simulink model "main_sim"  (R2024b)
settings: Solver=ode15s  StartTime=0.0  StopTime=t_sim  RelTol=1e-3
InitFcn:
  | rng('shuffle');
values from neighbouring files (symbols this model uses):
  accel_bias_instability = 9.8*40e-6    (= 0.000392)    [main.m]
  accel_PSD = accel_noise_power^2    (= 4.70596e-07)    [main.m]
  EA_0 = deg2rad([-2.83 -9.89 149]')    [Choi_SimulinkScript.m]    (also in SADS_UKF_Script.m = deg2rad([10 3 6]'); main.m = deg2rad([-8, 15, 0]'))
  g_N = [0 0 -9.81]    [Choi_SimulinkScript.m]    (also in SADS_UKF_Script.m; main.m)
  gyro_bias_instability = (pi/180)*(6/3600)    (= 2.90888208666e-05)    [main.m]
  gyro_PSD = gyro_noise_power^2    (= 2.74155703361e-09)    [main.m]
  J_0 = [1.815  -0.014 0.004 ... (first row only)    [Choi_SimulinkScript.m]    (also in LSR_sim.m = S.J_0; main.m)
  K_I = gainScale*5    (= 2.5)    [Choi_SimulinkScript.m]    (also in main.m)
  K_omega = gainScale*1    (= 0.5)    [Choi_SimulinkScript.m]    (also in main.m)
  k_p = 0.001    [Choi_SimulinkScript.m]
  K_q = gainScale*1    (= 0.5)    [Choi_SimulinkScript.m]    (also in main.m)
  L = [sample_time*(J_0\eye(3)), zeros(3,4) ... (first row only)    [main.m]
  m_s = 29    [Choi_SimulinkScript.m]    (also in LSR_sim.m = S.m_s; SADS_UKF_Script.m; main.m)
  omega_0 = [0 0.00 0.06]'    [Choi_SimulinkScript.m]    (also in SADS_UKF_Script.m = [0 0.00 0.05]'; main.m)
  P_0 = diag([1e-6 1e-6 1e-6 1e-6 1e-6 1e-6 1e-6 1e-6])    [SADS_UKF_Script.m]    (also in main.m = diag([1e-6 1e-6 1e-6 1e-6 1e-6 1e-6 1e-6]))
  Q = diag([5e-5 5e-5 5e-5 4e-12 4e-12 4e-12 4e-12 5e-6])    [SADS_UKF_Script.m]    (also in main.m = diag([5e-5 5e-5 5e-5 4e-11 4e-11 4e-11 4e-11]))
  q_0 = eul2quat(EA_0',"XYZ")'    [Choi_SimulinkScript.m]    (also in SADS_UKF_Script.m; main.m)
  q_d = [1 0 0 0]'    [Choi_SimulinkScript.m]    (also in main.m)
  R = diag([0.005 0.005 0.005].^2)    [SADS_UKF_Script.m]    (also in main.m)
  r_0 = [4*10^-3, 2*10^-3 ,-2*10^-2]'    [Choi_SimulinkScript.m]    (also in SADS_UKF_Script.m = [-0.003 0.006 -0.010]'; main.m = [0 0 0]')
  r_hat_0 = [0 0 -0.1]'    [Choi_SimulinkScript.m]
  r_imu_b = [0.1524, 0, 0.1524]    [main.m]
  sample_time = 1/sample_rate    (= 0.04)    [SADS_UKF_Script.m]    (also in main.m = 0.1)
  x_0 = [omega_0; q_0; 0]    [SADS_UKF_Script.m]
undefined symbols (not defined in the file or in its folder): A_pinv, A_truth, DiscIntNeverNeededParam, Gamma, gamma, h_d_amp, h_d_amp_LSR, h_d_period, h_d_period_LSR, h_d_phase, h_d_phase_LSR, H_ukf, I_wheel, Kappa, Kd_FSFB, Kp_FSFB, P_0_ukf, Q_ukf, R_ukf, tau_delay, x_0_ukf
libraries: simulink x6, matrix_library x4, sharedtransform x2, simulink_extras x1
settings Model: Creator=camer  LastModifiedBy=camer

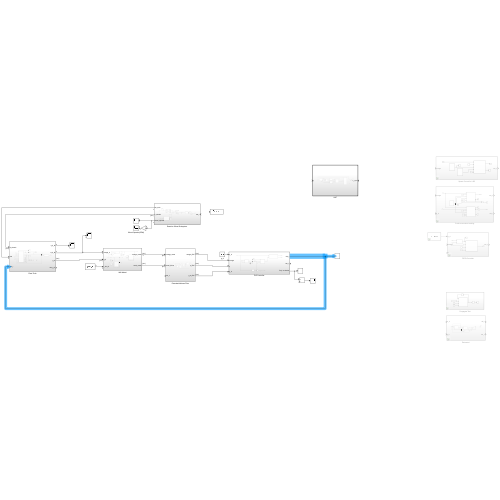
[thumbnail: Simulink's stored preview of the top-level diagram]
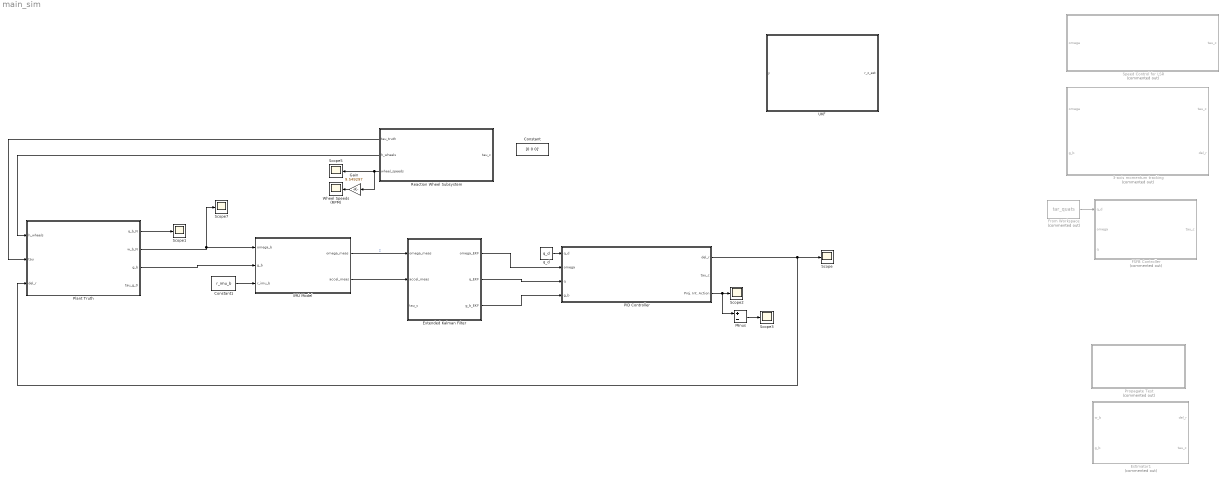
== system main_sim ==
  3-axis momentum tracking : Subsystem  Commented=on
  Constant : Constant  Value=[0 0 0]'
  Constant1 : Constant  Value=r_imu_b
  Estimator1 : Subsystem  Commented=on
  Extended Kalman Filter : Subsystem
  FSFB Controller : Subsystem  Commented=on
  From Workspace : FromWorkspace  Commented=on  VariableName=tar_quats
  Gain : Gain  Gain=9.549297
  IMU Model : Subsystem
  Minus : Sum  Inputs=+-
  PID Controller : Subsystem
  Plant Truth : Subsystem
  Propagate Test : Subsystem  Commented=on
  Reaction Wheel Subsystem : Subsystem
  Scope{,1..3,5,7} (6 alike) : Scope
  Speed Control for LSR : Subsystem  Commented=on
  UKF : Subsystem  TreatAsAtomicUnit=on
  Wheel Speeds (RPM) : Scope
  q_d : Constant  Value=q_d
  wires:
  IMU Model/1(omega_meas) -> Extended Kalman Filter/1(omega_meas)  "z"
  Constant1/1 -> IMU Model/3(r_imu_b)
  IMU Model/2(accel_meas) -> Extended Kalman Filter/2(accel_meas)
  From Workspace/1 -> FSFB Controller/1(q_d)
  Plant Truth/1(q_b_N) -> Scope1/1
  Reaction Wheel Subsystem/3(wheel_speeds) -> Scope5/1, Gain/1
  Reaction Wheel Subsystem/1(tau_truth) -> Plant Truth/2(tau)
  Plant Truth/2(w_b_N) -> Scope7/1, IMU Model/1(omega_b)
  Plant Truth/3(g_b) -> IMU Model/2(g_b)
  Reaction Wheel Subsystem/2(h_wheels) -> Plant Truth/1(h_wheels)
  Gain/1 -> Wheel Speeds (RPM)/1
  PID Controller/1(del_r) -> Plant Truth/3(del_r), Scope/1
  PID Controller/3(Proj. Int. Action) -> Minus/1, Scope2/1
  Minus/1 -> Scope3/1
  q_d/1 -> PID Controller/1(q_d)
  Extended Kalman Filter/1(omega_EKF) -> PID Controller/2(omega)
  Extended Kalman Filter/2(q_EKF) -> PID Controller/3(q)
  Extended Kalman Filter/3(g_b_EKF) -> PID Controller/4(g_b)

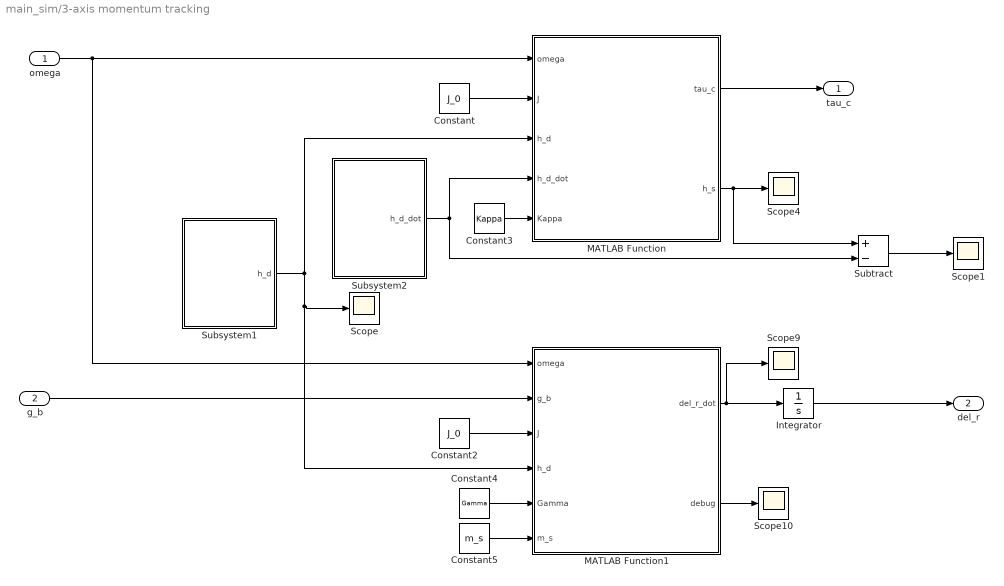
== system main_sim/3-axis momentum tracking ==
  omega : Inport
  g_b : Inport  Port=2
  Constant : Constant  Value=J_0
  Constant2 : Constant  Value=J_0
  Constant3 : Constant  Value=Kappa
  Constant4 : Constant  Value=Gamma
  Constant5 : Constant  Value=m_s
  Integrator : Integrator  InitialCondition=[0 0 0]'
  MATLAB Function : MATLAB Function  TreatAsAtomicUnit=on
  MATLAB Function1 : MATLAB Function  TreatAsAtomicUnit=on
  Scope{,1,4,9..10} (5 alike) : Scope
  Subsystem1 : Subsystem
  Subsystem2 : Subsystem
  Subtract : Sum  Inputs=+-
  tau_c : Outport
  del_r : Outport  Port=2
  wires:
  g_b/1 -> MATLAB Function1/2(g_b)
  Constant/1 -> MATLAB Function/2(J)
  MATLAB Function1/2(debug) -> Scope10/1
  MATLAB Function1/1(del_r_dot) -> Integrator/1, Scope9/1
  Constant2/1 -> MATLAB Function1/3(J)
  MATLAB Function/1(tau_c) -> tau_c/1
  MATLAB Function/2(h_s) -> Subtract/1, Scope4/1
  Constant4/1 -> MATLAB Function1/5(Gamma)
  Constant5/1 -> MATLAB Function1/6(m_s)
  omega/1 -> MATLAB Function1/1(omega), MATLAB Function/1(omega)
  Constant3/1 -> MATLAB Function/5(Kappa)
  Integrator/1 -> del_r/1
  Subsystem2/1(h_d_dot) -> Subtract/2, MATLAB Function/4(h_d_dot)
  Subsystem1/1(h_d) -> Scope/1, MATLAB Function1/4(h_d), MATLAB Function/3(h_d)
  Subtract/1 -> Scope1/1

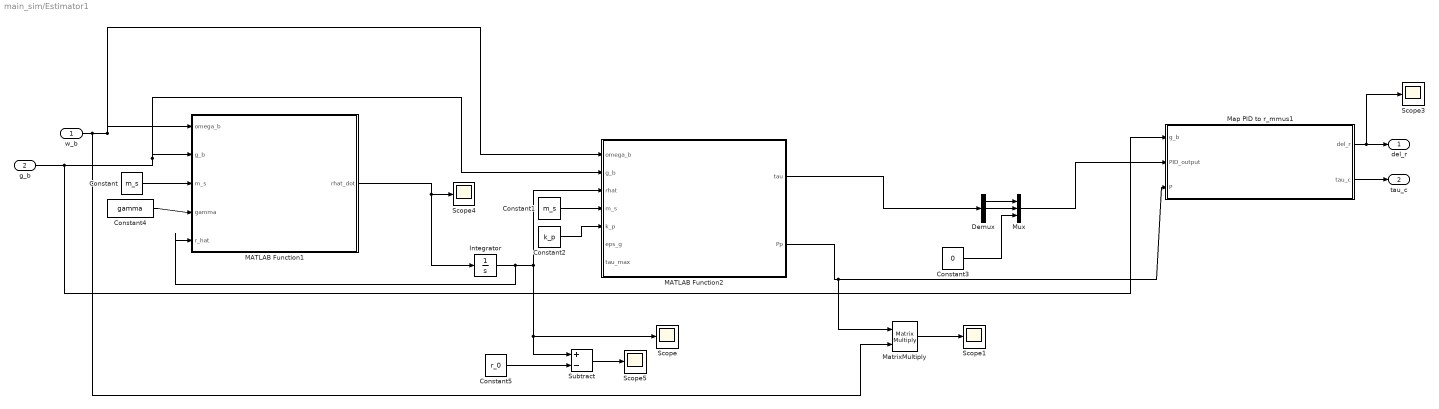
== system main_sim/Estimator1 ==
  w_b : Inport
  g_b : Inport  Port=2
  Constant : Constant  Value=m_s
  Constant1 : Constant  Value=m_s
  Constant2 : Constant  Value=k_p
  Constant3 : Constant  Value=0
  Constant4 : Constant  Value=gamma
  Constant5 : Constant  Value=r_0
  Demux : Demux  Outputs=3
  Integrator : Integrator  InitialCondition=r_hat_0
  MATLAB Function1 : MATLAB Function  TreatAsAtomicUnit=on
  MATLAB Function2 : MATLAB Function  TreatAsAtomicUnit=on
  Map PID to r_mmus1 : Subsystem
  MatrixMultiply : Product  Multiplication=Matrix(*)
  Mux : Mux  Inputs=3
  Scope{,1,3..5} (5 alike) : Scope
  Subtract : Sum  Inputs=+-
  del_r : Outport
  tau_c : Outport  Port=2
  wires:
  g_b/1 -> Map PID to r_mmus1/1(g_b), MATLAB Function2/2(g_b), MATLAB Function1/2(g_b)
  Constant/1 -> MATLAB Function1/3(m_s)
  MATLAB Function1/1(rhat_dot) -> Scope4/1, Integrator/1
  Integrator/1 -> MATLAB Function1/5(r_hat), Subtract/1, Scope/1, MATLAB Function2/3(rhat)
  Constant1/1 -> MATLAB Function2/4(m_s)
  Constant2/1 -> MATLAB Function2/5(k_p)
  MATLAB Function2/1(tau) -> Demux/1
  Demux/1 -> Mux/1
  Constant3/1 -> Mux/3
  Demux/2 -> Mux/2
  Map PID to r_mmus1/1(del_r) -> Scope3/1, del_r/1
  w_b/1 -> MatrixMultiply/2, MATLAB Function1/1(omega_b), MATLAB Function2/1(omega_b)
  Constant4/1 -> MATLAB Function1/4(gamma)
  Map PID to r_mmus1/2(tau_c) -> tau_c/1
  MATLAB Function2/2(Pp) -> MatrixMultiply/1, Map PID to r_mmus1/3(P)
  MatrixMultiply/1 -> Scope1/1
  Constant5/1 -> Subtract/2
  Subtract/1 -> Scope5/1
  Mux/1 -> Map PID to r_mmus1/2(PID_output)

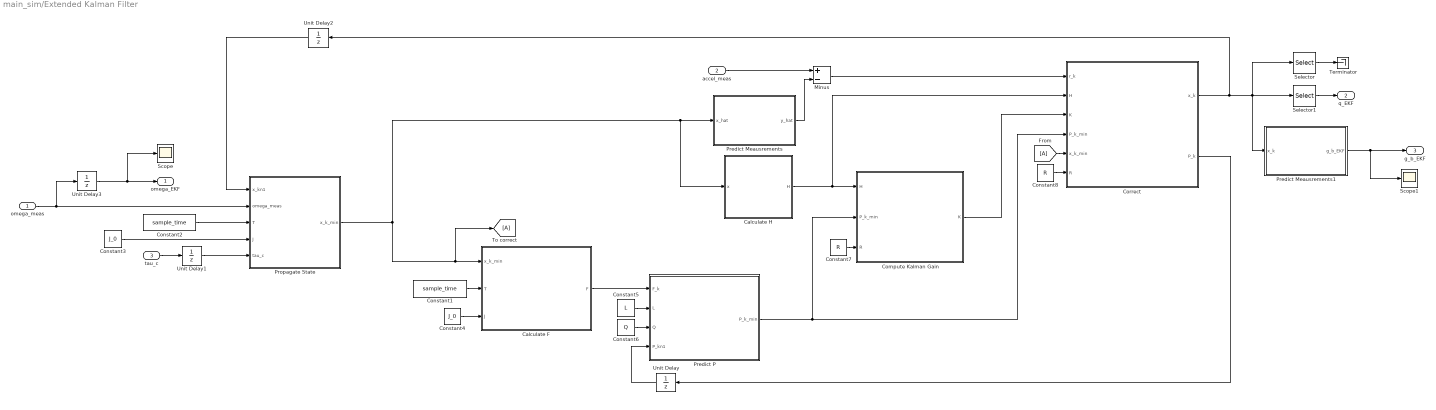
== system main_sim/Extended Kalman Filter ==
  omega_meas : Inport
  accel_meas : Inport  Port=2
  tau_c : Inport  Port=3
  Calculate F : MATLAB Function  TreatAsAtomicUnit=on
  Calculate H : MATLAB Function  TreatAsAtomicUnit=on
  Compute Kalman Gain : MATLAB Function  TreatAsAtomicUnit=on
  Constant1 : Constant  Value=sample_time
  Constant2 : Constant  Value=sample_time
  Constant3 : Constant  Value=J_0
  Constant4 : Constant  Value=J_0
  Constant5 : Constant  Value=L
  Constant6 : Constant  Value=Q
  Constant7 : Constant  Value=R
  Constant8 : Constant  Value=R
  Correct : MATLAB Function  TreatAsAtomicUnit=on
  From : From
  Minus : Sum  Inputs=+-
  Predict Meausrements : MATLAB Function  TreatAsAtomicUnit=on
  Predict Meausrements1 : MATLAB Function  TreatAsAtomicUnit=on
  Predict P : MATLAB Function  TreatAsAtomicUnit=on
  Propagate State : MATLAB Function  TreatAsAtomicUnit=on
  Scope : Scope
  Scope1 : Scope
  Selector : Selector  InputPortWidth=7  IndexOptions=Index vector (dialog)  Indices=[1 2 3]  OutputSizes=1
  Selector1 : Selector  InputPortWidth=7  IndexOptions=Index vector (dialog)  Indices=[4 5 6 7]  OutputSizes=1
  Terminator : Terminator
  To correct : Goto
  Unit Delay : UnitDelay  InitialCondition=P_0  SampleTime=sample_time  HasFrameUpgradeWarning=on
  Unit Delay1 : UnitDelay  InitialCondition=[0 0 0]'  SampleTime=-1  HasFrameUpgradeWarning=on
  Unit Delay2 : UnitDelay  InitialCondition=x_0  SampleTime=sample_time  HasFrameUpgradeWarning=on
  Unit Delay3 : UnitDelay  InitialCondition=[0 0 0]'  SampleTime=-1  HasFrameUpgradeWarning=on
  omega_EKF : Outport
  q_EKF : Outport  Port=2
  g_b_EKF : Outport  Port=3
  wires:
  Constant3/1 -> Propagate State/4(J)
  Propagate State/1(x_k_min) -> Calculate H/1(x), Predict Meausrements/1(x_hat), To correct/1, Calculate F/1(x_k_min)
  Unit Delay2/1 -> Propagate State/1(x_kn1)
  Constant2/1 -> Propagate State/3(T)
  Constant1/1 -> Calculate F/2(T)
  Constant4/1 -> Calculate F/3(J)
  Calculate F/1(F) -> Predict P/1(F_k)
  Unit Delay/1 -> Predict P/4(P_kn1)
  Constant5/1 -> Predict P/2(L)
  Constant6/1 -> Predict P/3(Q)
  accel_meas/1 -> Minus/1
  Predict Meausrements/1(y_hat) -> Minus/2
  Minus/1 -> Correct/1(r_k)
  Calculate H/1(H) -> Correct/2(H), Compute Kalman Gain/1(H)
  Predict P/1(P_k_min) -> Compute Kalman Gain/2(P_k_min), Correct/4(P_k_min)
  Constant7/1 -> Compute Kalman Gain/3(R)
  Compute Kalman Gain/1(K) -> Correct/3(K)
  Constant8/1 -> Correct/6(R)
  Correct/2(P_k) -> Unit Delay/1
  From/1 -> Correct/5(x_k_min)
  omega_meas/1 -> Propagate State/2(omega_meas), Unit Delay3/1
  Correct/1(x_k) -> Selector/1, Selector1/1, Predict Meausrements1/1(x_k), Unit Delay2/1
  Predict Meausrements1/1(g_b_EKF) -> Scope1/1, g_b_EKF/1
  Selector/1 -> Terminator/1
  Selector1/1 -> q_EKF/1
  tau_c/1 -> Unit Delay1/1
  Unit Delay1/1 -> Propagate State/5(tau_c)
  Unit Delay3/1 -> Scope/1, omega_EKF/1

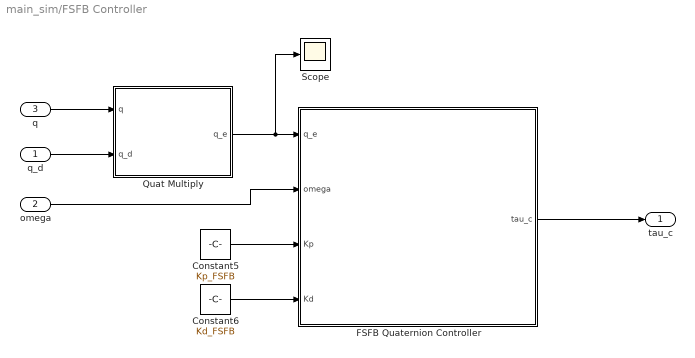
== system main_sim/FSFB Controller ==
  q_d : Inport
  omega : Inport  Port=2
  q : Inport  Port=3
  Constant5 : Constant  Value=Kp_FSFB
  Constant6 : Constant  Value=Kd_FSFB
  FSFB Quaternion Controller : MATLAB Function  TreatAsAtomicUnit=on
  Quat Multiply : MATLAB Function  TreatAsAtomicUnit=on
  Scope : Scope
  tau_c : Outport
  wires:
  Constant6/1 -> FSFB Quaternion Controller/4(Kd)
  FSFB Quaternion Controller/1(tau_c) -> tau_c/1
  omega/1 -> FSFB Quaternion Controller/2(omega)
  Constant5/1 -> FSFB Quaternion Controller/3(Kp)
  q_d/1 -> Quat Multiply/2(q_d)
  Quat Multiply/1(q_e) -> Scope/1, FSFB Quaternion Controller/1(q_e)
  q/1 -> Quat Multiply/1(q)

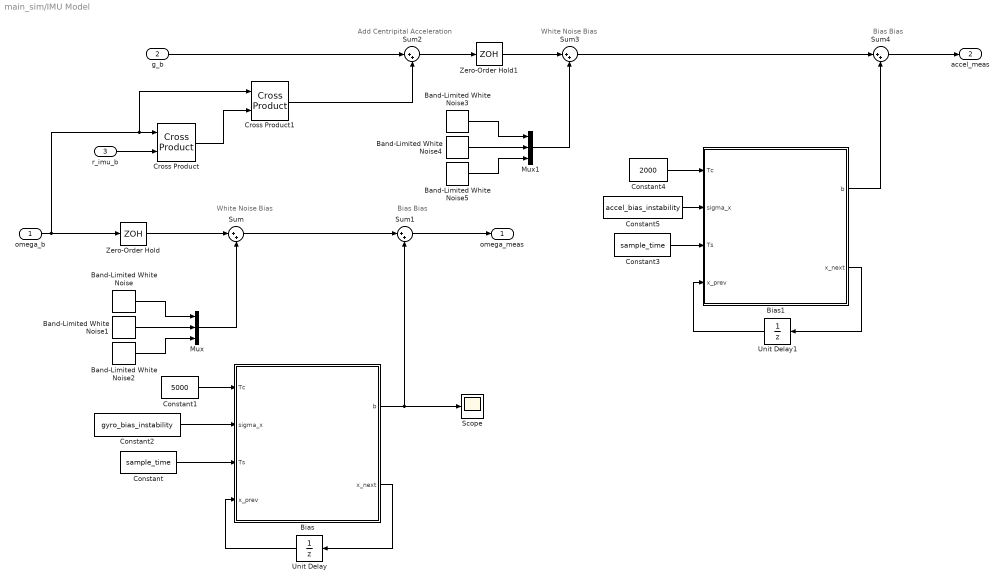
== system main_sim/IMU Model ==
  note: Add Centripital Acceleration
  note: Bias
      | Bias
  note: Bias
      | Bias
  note: White Noise
      | Bias
  note: White Noise
      | Bias
  omega_b : Inport
  g_b : Inport  Port=2
  r_imu_b : Inport  Port=3
  Band-Limited White Noise : simulink/Sources/Band-Limited White Noise  Cov=[gyro_PSD]  Ts=sample_time  seed=[23341]
  Band-Limited White Noise1 : simulink/Sources/Band-Limited White Noise  Cov=[gyro_PSD]  Ts=sample_time  seed=[23141]
  Band-Limited White Noise2 : simulink/Sources/Band-Limited White Noise  Cov=[gyro_PSD]  Ts=sample_time  seed=[35163]
  Band-Limited White Noise3 : simulink/Sources/Band-Limited White Noise  Cov=[accel_PSD]  Ts=sample_time  seed=[23341]
  Band-Limited White Noise4 : simulink/Sources/Band-Limited White Noise  Cov=[accel_PSD]  Ts=sample_time  seed=[23141]
  Band-Limited White Noise5 : simulink/Sources/Band-Limited White Noise  Cov=[accel_PSD]  Ts=sample_time  seed=[35163]
  Bias : MATLAB Function  TreatAsAtomicUnit=on
  Bias1 : MATLAB Function  TreatAsAtomicUnit=on
  Constant : Constant  Value=sample_time
  Constant1 : Constant  Value=5000
  Constant2 : Constant  Value=gyro_bias_instability
  Constant3 : Constant  Value=sample_time
  Constant4 : Constant  Value=2000
  Constant5 : Constant  Value=accel_bias_instability
  Cross Product : matrix_library/Cross Product
  Cross Product1 : matrix_library/Cross Product
  Mux : Mux  Inputs=3
  Mux1 : Mux  Inputs=3
  Scope : Scope
  Sum{,1..4} (5 alike) : Sum  Inputs=|++
  Unit Delay : UnitDelay  InitialCondition=gyro_bias_instability*randn(3,1)  SampleTime=sample_time  HasFrameUpgradeWarning=on
  Unit Delay1 : UnitDelay  InitialCondition=accel_bias_instability*randn(3,1)  SampleTime=sample_time  HasFrameUpgradeWarning=on
  Zero-Order Hold : ZeroOrderHold  SampleTime=sample_time
  Zero-Order Hold1 : ZeroOrderHold  SampleTime=sample_time
  omega_meas : Outport
  accel_meas : Outport  Port=2
  wires:
  Band-Limited White Noise1/1 -> Mux/2
  Band-Limited White Noise/1 -> Mux/1
  Band-Limited White Noise2/1 -> Mux/3
  Mux/1 -> Sum/2
  Zero-Order Hold/1 -> Sum/1
  Bias/2(x_next) -> Unit Delay/1
  Sum1/1 -> omega_meas/1
  Bias/1(b) -> Scope/1, Sum1/2
  Unit Delay/1 -> Bias/4(x_prev)
  Constant/1 -> Bias/3(Ts)
  Constant1/1 -> Bias/1(Tc)
  Constant2/1 -> Bias/2(sigma_x)
  Sum/1 -> Sum1/1
  r_imu_b/1 -> Cross Product/2
  Cross Product/1 -> Cross Product1/2
  Cross Product1/1 -> Sum2/2
  g_b/1 -> Sum2/1
  Sum2/1 -> Zero-Order Hold1/1
  Band-Limited White Noise5/1 -> Mux1/3
  Band-Limited White Noise4/1 -> Mux1/2
  Band-Limited White Noise3/1 -> Mux1/1
  Mux1/1 -> Sum3/2
  omega_b/1 -> Zero-Order Hold/1, Cross Product1/1, Cross Product/1
  Zero-Order Hold1/1 -> Sum3/1
  Unit Delay1/1 -> Bias1/4(x_prev)
  Bias1/1(b) -> Sum4/2
  Constant3/1 -> Bias1/3(Ts)
  Constant4/1 -> Bias1/1(Tc)
  Bias1/2(x_next) -> Unit Delay1/1
  Constant5/1 -> Bias1/2(sigma_x)
  Sum3/1 -> Sum4/1
  Sum4/1 -> accel_meas/1

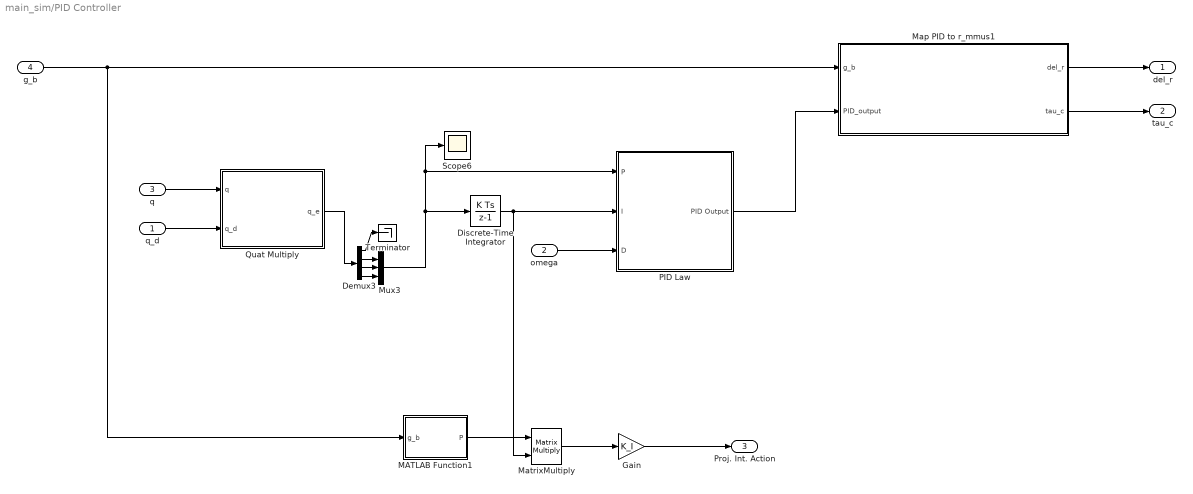
== system main_sim/PID Controller ==
  q_d : Inport
  omega : Inport  Port=2
  q : Inport  Port=3
  g_b : Inport  Port=4
  Demux3 : Demux
  Discrete-Time Integrator : DiscreteIntegrator  InitialCondition=[0,0,0]'  SampleTime=sample_time  ICPrevOutput=DiscIntNeverNeededParam  ICPrevScaledInput=DiscIntNeverNeededParam
  Gain : Gain  Gain=K_I
  MATLAB Function1 : MATLAB Function  TreatAsAtomicUnit=on
  Map PID to r_mmus1 : Subsystem
  MatrixMultiply : Product  Multiplication=Matrix(*)
  Mux3 : Mux  Inputs=3
  PID Law : Subsystem
  Quat Multiply : MATLAB Function  TreatAsAtomicUnit=on
  Scope6 : Scope
  Terminator : Terminator
  del_r : Outport
  tau_c : Outport  Port=2
  Proj. Int. Action : Outport  Port=3
  wires:
  Mux3/1 -> Discrete-Time Integrator/1, Scope6/1, PID Law/1(P)
  Demux3/4 -> Mux3/3
  Demux3/3 -> Mux3/2
  Demux3/2 -> Mux3/1
  q/1 -> Quat Multiply/1(q)
  Discrete-Time Integrator/1 -> MatrixMultiply/2, PID Law/2(I)
  Quat Multiply/1(q_e) -> Demux3/1
  PID Law/1(PID Output) -> Map PID to r_mmus1/2(PID_output)
  q_d/1 -> Quat Multiply/2(q_d)
  Demux3/1 -> Terminator/1
  omega/1 -> PID Law/3(D)
  g_b/1 -> MATLAB Function1/1(g_b), Map PID to r_mmus1/1(g_b)
  Map PID to r_mmus1/1(del_r) -> del_r/1
  Map PID to r_mmus1/2(tau_c) -> tau_c/1
  MATLAB Function1/1(P) -> MatrixMultiply/1
  MatrixMultiply/1 -> Gain/1
  Gain/1 -> Proj. Int. Action/1

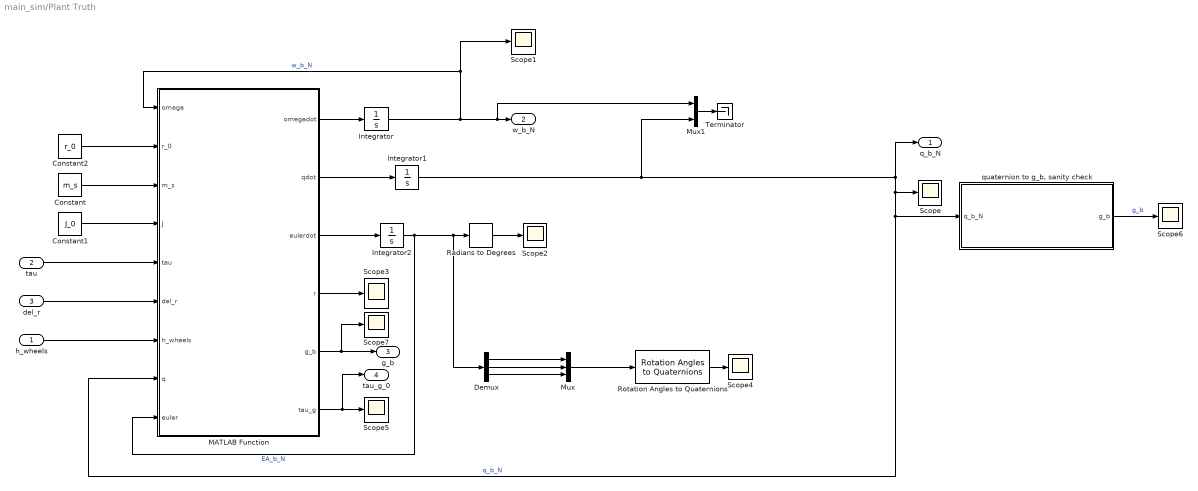
== system main_sim/Plant Truth ==
  h_wheels : Inport
  tau : Inport  Port=2
  del_r : Inport  Port=3
  Constant : Constant  Value=m_s
  Constant1 : Constant  Value=J_0
  Constant2 : Constant  Value=r_0
  Demux : Demux  Outputs=3
  Integrator : Integrator  InitialCondition=omega_0
  Integrator1 : Integrator  InitialCondition=q_0
  Integrator2 : Integrator  InitialCondition=EA_0
  MATLAB Function : MATLAB Function  TreatAsAtomicUnit=on
  Mux : Mux  Inputs=3
  Mux1 : Mux  Inputs=2
  Radians to Degrees : simulink_extras/Transformations/Radians to Degrees
  Rotation Angles to Quaternions : sharedtransform/Rotation Angles to Quaternions  rotationOrder=XYZ  aMode=aMode
  Scope{,1..7} (8 alike) : Scope
  Terminator : Terminator
  "quaternion to g_b, sanity check" : Subsystem
  q_b_N : Outport
  w_b_N : Outport  Port=2
  g_b : Outport  Port=3
  tau_g_0 : Outport  Port=4
  wires:
  MATLAB Function/4(r) -> Scope3/1
  Integrator/1 -> Scope1/1, MATLAB Function/1(omega), Mux1/1, w_b_N/1  "w_b_N"
  Constant1/1 -> MATLAB Function/4(J)
  Constant2/1 -> MATLAB Function/2(r_0)
  Constant/1 -> MATLAB Function/3(m_s)
  tau/1 -> MATLAB Function/5(tau)
  Integrator1/1 -> Mux1/2, q_b_N/1, Scope/1, MATLAB Function/8(q), "quaternion to g_b, sanity check"/1(q_b_N)  "q_b_N"
  MATLAB Function/2(qdot) -> Integrator1/1
  MATLAB Function/1(omegadot) -> Integrator/1
  del_r/1 -> MATLAB Function/6(del_r)
  "quaternion to g_b, sanity check"/1(g_b) -> Scope6/1  "g_b"
  MATLAB Function/3(eulerdot) -> Integrator2/1
  Integrator2/1 -> Radians to Degrees/1, Demux/1, MATLAB Function/9(euler)  "EA_b_N"
  Demux/2 -> Mux/2
  Demux/1 -> Mux/1
  Mux/1 -> Rotation Angles to Quaternions/1
  Rotation Angles to Quaternions/1 -> Scope4/1
  MATLAB Function/5(g_b) -> Scope7/1, g_b/1
  Mux1/1 -> Terminator/1
  MATLAB Function/6(tau_g) -> tau_g_0/1, Scope5/1
  Radians to Degrees/1 -> Scope2/1
  h_wheels/1 -> MATLAB Function/7(h_wheels)
  Demux/3 -> Mux/3

== system main_sim/Propagate Test ==
  Constant2 : Constant  Value=sample_time
  Constant3 : Constant  Value=J_0
  Constant5 : Constant  Value=m_s
  Propagate State : MATLAB Function  TreatAsAtomicUnit=on
  Scope3 : Scope
  Selector : Selector  InputPortWidth=8  IndexOptions=Index vector (dialog)  Indices=[4 5 6 7]  OutputSizes=1
  Unit Delay2 : UnitDelay  InitialCondition=[omega_0; q_0; r_0(3)];  SampleTime=sample_time  HasFrameUpgradeWarning=on
  wires:
  Constant5/1 -> Propagate State/4(m_s)
  Constant3/1 -> Propagate State/3(J)
  Propagate State/1(x_k_i) -> Selector/1, Unit Delay2/1  "x_k_i"
  Unit Delay2/1 -> Propagate State/1(x_kn1_i)
  Selector/1 -> Scope3/1
  Constant2/1 -> Propagate State/2(T)

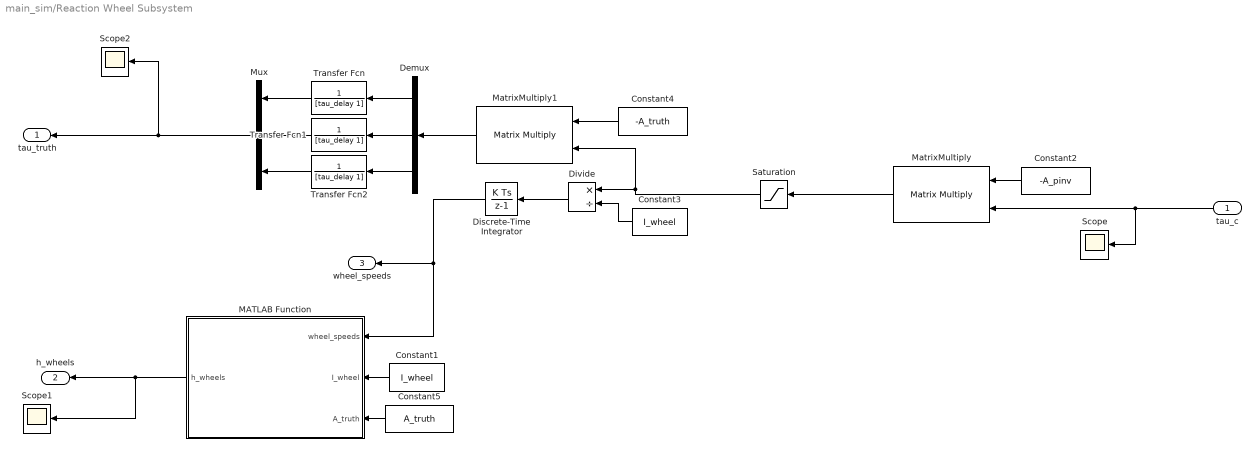
== system main_sim/Reaction Wheel Subsystem ==
  tau_c : Inport
  Constant1 : Constant  Value=I_wheel
  Constant2 : Constant  Value=-A_pinv
  Constant3 : Constant  Value=I_wheel
  Constant4 : Constant  Value=-A_truth
  Constant5 : Constant  Value=A_truth
  Demux : Demux  Outputs=3
  Discrete-Time Integrator : DiscreteIntegrator  SampleTime=sample_time  ICPrevOutput=DiscIntNeverNeededParam  ICPrevScaledInput=DiscIntNeverNeededParam
  Divide : Product  Inputs=*/
  MATLAB Function : MATLAB Function  TreatAsAtomicUnit=on
  MatrixMultiply : Product  Multiplication=Matrix(*)
  MatrixMultiply1 : Product  Multiplication=Matrix(*)
  Mux : Mux  Inputs=3
  Saturation : Saturate  UpperLimit=0.1  LowerLimit=-0.1
  Scope : Scope
  Scope1 : Scope
  Scope2 : Scope
  Transfer Fcn : TransferFcn  Denominator=[tau_delay 1]
  Transfer Fcn1 : TransferFcn  Denominator=[tau_delay 1]
  Transfer Fcn2 : TransferFcn  Denominator=[tau_delay 1]
  tau_truth : Outport
  h_wheels : Outport  Port=2
  wheel_speeds : Outport  Port=3
  wires:
  Discrete-Time Integrator/1 -> MATLAB Function/1(wheel_speeds), wheel_speeds/1
  Constant4/1 -> MatrixMultiply1/1
  MatrixMultiply/1 -> Saturation/1
  Constant3/1 -> Divide/2
  tau_c/1 -> Scope/1, MatrixMultiply/2
  Constant2/1 -> MatrixMultiply/1
  Divide/1 -> Discrete-Time Integrator/1
  Demux/1 -> Transfer Fcn/1
  Demux/2 -> Transfer Fcn1/1
  Demux/3 -> Transfer Fcn2/1
  Transfer Fcn/1 -> Mux/1
  Transfer Fcn1/1 -> Mux/2
  Transfer Fcn2/1 -> Mux/3
  MatrixMultiply1/1 -> Demux/1
  Mux/1 -> Scope2/1, tau_truth/1
  MATLAB Function/1(h_wheels) -> Scope1/1, h_wheels/1
  Constant1/1 -> MATLAB Function/2(I_wheel)
  Constant5/1 -> MATLAB Function/3(A_truth)
  Saturation/1 -> MatrixMultiply1/2, Divide/1

== system main_sim/Speed Control for LSR ==
  omega : Inport
  Constant : Constant  Value=J_0
  Constant3 : Constant  Value=Kappa
  MATLAB Function : MATLAB Function  TreatAsAtomicUnit=on
  Scope : Scope
  Scope4 : Scope
  Subsystem1 : Subsystem
  Subsystem2 : Subsystem
  tau_c : Outport
  wires:
  Constant/1 -> MATLAB Function/2(J)
  MATLAB Function/1(tau_c) -> tau_c/1
  MATLAB Function/2(h_s) -> Scope4/1
  omega/1 -> MATLAB Function/1(omega)
  Constant3/1 -> MATLAB Function/5(Kappa)
  Subsystem2/1(h_d_dot) -> MATLAB Function/4(h_d_dot)
  Subsystem1/1(h_d) -> Scope/1, MATLAB Function/3(h_d)

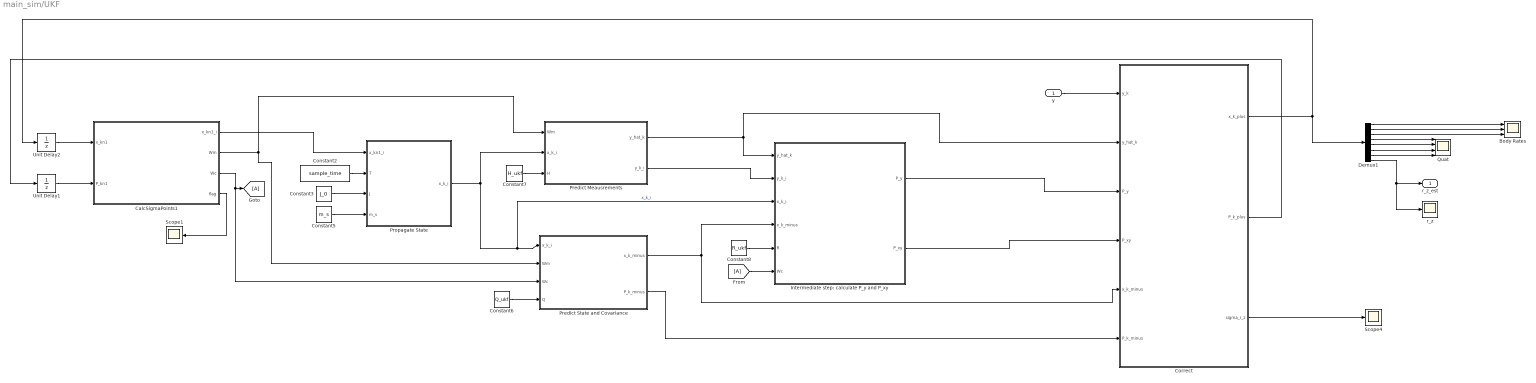
== system main_sim/UKF ==
  y : Inport
  Body Rates : Scope  NumInputPorts=3
  CalcSigmaPoints1 : MATLAB Function  TreatAsAtomicUnit=on
  Constant2 : Constant  Value=sample_time
  Constant3 : Constant  Value=J_0
  Constant5 : Constant  Value=m_s
  Constant6 : Constant  Value=Q_ukf
  Constant7 : Constant  Value=H_ukf
  Constant8 : Constant  Value=R_ukf
  Correct : MATLAB Function  TreatAsAtomicUnit=on
  Demux1 : Demux  Outputs=8
  From : From
  Goto : Goto
  Intermediate step: calculate P_y and P_xy : MATLAB Function  TreatAsAtomicUnit=on
  Predict Meausrements : MATLAB Function  TreatAsAtomicUnit=on
  Predict State and Covariance : MATLAB Function  TreatAsAtomicUnit=on
  Propagate State : MATLAB Function  TreatAsAtomicUnit=on
  Quat : Scope  NumInputPorts=4
  Scope1 : Scope
  Scope4 : Scope
  Unit Delay1 : UnitDelay  InitialCondition=P_0_ukf  SampleTime=sample_time  HasFrameUpgradeWarning=on
  Unit Delay2 : UnitDelay  InitialCondition=x_0_ukf  SampleTime=sample_time  HasFrameUpgradeWarning=on
  r_z : Scope
  r_z_est : Outport
  wires:
  CalcSigmaPoints1/1(x_kn1_i) -> Propagate State/1(x_kn1_i)
  Constant3/1 -> Propagate State/3(J)
  Constant2/1 -> Propagate State/2(T)
  Propagate State/1(x_k_i) -> Intermediate step: calculate P_y and P_xy/3(x_k_i), Predict State and Covariance/1(x_k_i), Predict Meausrements/2(x_k_i)  "x_k_i"
  Constant6/1 -> Predict State and Covariance/4(Q)
  Predict State and Covariance/1(x_k_minus) -> Intermediate step: calculate P_y and P_xy/4(x_k_minus), Correct/5(x_k_minus)
  Predict Meausrements/1(y_hat_k) -> Intermediate step: calculate P_y and P_xy/1(y_hat_k), Correct/2(y_hat_k)
  Predict State and Covariance/2(P_k_minus) -> Correct/6(P_k_minus)
  Constant7/1 -> Predict Meausrements/3(H)
  Predict Meausrements/2(y_k_i) -> Intermediate step: calculate P_y and P_xy/2(y_k_i)
  Constant8/1 -> Intermediate step: calculate P_y and P_xy/5(R)
  y/1 -> Correct/1(y_k)
  Intermediate step: calculate P_y and P_xy/1(P_y) -> Correct/3(P_y)
  Intermediate step: calculate P_y and P_xy/2(P_xy) -> Correct/4(P_xy)
  Correct/2(P_k_plus) -> Unit Delay1/1
  Correct/1(x_k_plus) -> Demux1/1, Unit Delay2/1
  Unit Delay1/1 -> CalcSigmaPoints1/2(P_kn1)
  Unit Delay2/1 -> CalcSigmaPoints1/1(x_kn1)
  CalcSigmaPoints1/2(Wm) -> Predict State and Covariance/2(Wm), Predict Meausrements/1(Wm)
  CalcSigmaPoints1/3(Wc) -> Goto/1, Predict State and Covariance/3(Wc)
  From/1 -> Intermediate step: calculate P_y and P_xy/6(Wc)
  Demux1/5 -> Quat/2
  Demux1/4 -> Quat/1
  Demux1/6 -> Quat/3
  Demux1/7 -> Quat/4
  Constant5/1 -> Propagate State/4(m_s)
  Demux1/8 -> r_z_est/1, r_z/1
  Demux1/1 -> Body Rates/1
  Demux1/2 -> Body Rates/2
  Demux1/3 -> Body Rates/3
  Correct/3(sigma_r_z) -> Scope4/1
  CalcSigmaPoints1/4(flag) -> Scope1/1

== system main_sim/3-axis momentum tracking/Subsystem1 ==
  Mux1 : Mux  Inputs=3
  Sine Wave : Sin  Amplitude=h_d_amp(1)  Frequency=1/h_d_period(1)  Phase=h_d_phase(1)  SampleTime=0
  Sine Wave1 : Sin  Amplitude=h_d_amp(2)  Frequency=1/h_d_period(2)  Phase=h_d_phase(2)  SampleTime=0
  Sine Wave2 : Sin  Amplitude=h_d_amp(3)  Frequency=1/h_d_period(3)  Phase=h_d_phase(3)  SampleTime=0
  h_d : Outport
  wires:
  Sine Wave/1 -> Mux1/1
  Sine Wave2/1 -> Mux1/3
  Sine Wave1/1 -> Mux1/2
  Mux1/1 -> h_d/1

== system main_sim/3-axis momentum tracking/Subsystem2 ==
  Gain : Gain  Gain=1/h_d_period(1)
  Gain1 : Gain  Gain=1/h_d_period(2)
  Gain2 : Gain  Gain=1/h_d_period(3)
  Mux : Mux  Inputs=3
  Sine Wave3 : Sin  Amplitude=h_d_amp(1)  Frequency=1/h_d_period(1)  Phase=h_d_phase(1)-(pi/2)  SampleTime=0
  Sine Wave4 : Sin  Amplitude=h_d_amp(2)  Frequency=1/h_d_period(2)  Phase=h_d_phase(2)-(pi/2)  SampleTime=0
  Sine Wave5 : Sin  Amplitude=h_d_amp(3)  Frequency=1/h_d_period(3)  Phase=h_d_phase(3)-(pi/2)  SampleTime=0
  h_d_dot : Outport
  wires:
  Mux/1 -> h_d_dot/1
  Sine Wave5/1 -> Gain2/1
  Gain2/1 -> Mux/3
  Sine Wave3/1 -> Gain/1
  Sine Wave4/1 -> Gain1/1
  Gain1/1 -> Mux/2
  Gain/1 -> Mux/1

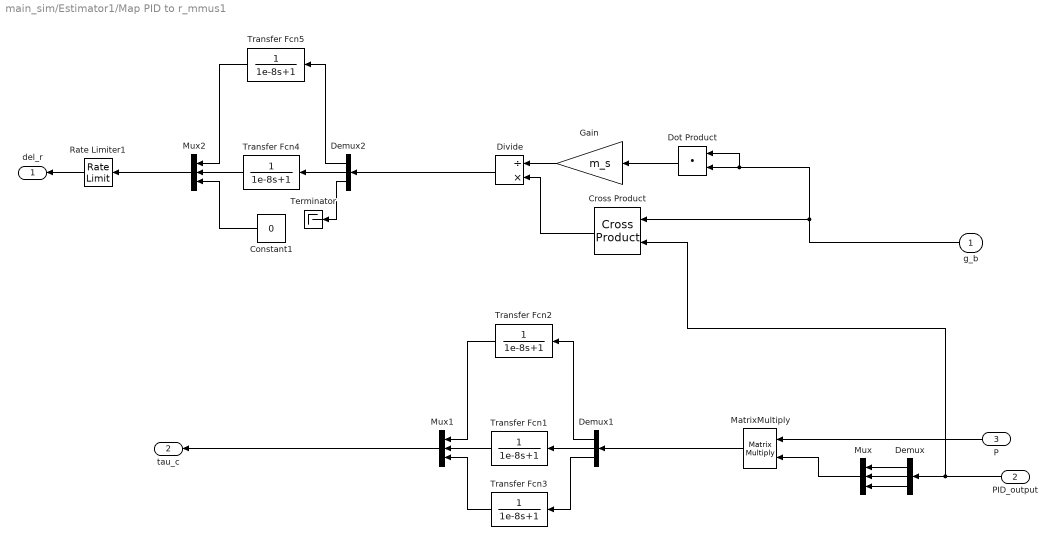
== system main_sim/Estimator1/Map PID to r_mmus1 ==
  g_b : Inport
  PID_output : Inport  Port=2
  P : Inport  Port=3
  Constant1 : Constant  Value=0
  Cross Product : matrix_library/Cross Product
  Demux : Demux  Outputs=3
  Demux1 : Demux  Outputs=3
  Demux2 : Demux  Outputs=3
  Divide : Product  Inputs=/*
  Dot Product : DotProduct  OutDataTypeStr=Inherit: Inherit via internal rule
  Gain : Gain  Gain=m_s
  MatrixMultiply : Product  Multiplication=Matrix(*)
  Mux : Mux  Inputs=3
  Mux1 : Mux  Inputs=3
  Mux2 : Mux  Inputs=3
  Rate Limiter1 : RateLimiter  RisingSlewLimit=0.030  FallingSlewLimit=-0.030  SampleTimeMode=inherited
  Terminator : Terminator
  Transfer Fcn{1..5} (5 alike) : TransferFcn  Denominator=[1e-8 1]
  del_r : Outport
  tau_c : Outport  Port=2
  wires:
  PID_output/1 -> Cross Product/2, Demux/1
  g_b/1 -> Dot Product/1, Dot Product/2, Cross Product/1
  Demux/2 -> Mux/2
  Demux/1 -> Mux/1
  Dot Product/1 -> Gain/1
  Gain/1 -> Divide/1
  Cross Product/1 -> Divide/2
  Transfer Fcn4/1 -> Mux2/2
  Constant1/1 -> Mux2/3
  Transfer Fcn5/1 -> Mux2/1
  Divide/1 -> Demux2/1
  Mux2/1 -> Rate Limiter1/1
  Demux2/2 -> Transfer Fcn4/1
  Demux2/1 -> Transfer Fcn5/1
  Rate Limiter1/1 -> del_r/1
  Demux2/3 -> Terminator/1
  Transfer Fcn3/1 -> Mux1/3
  Demux1/1 -> Transfer Fcn2/1
  Transfer Fcn1/1 -> Mux1/2
  Transfer Fcn2/1 -> Mux1/1
  Mux1/1 -> tau_c/1
  Demux1/3 -> Transfer Fcn3/1
  Demux1/2 -> Transfer Fcn1/1
  Demux/3 -> Mux/3
  P/1 -> MatrixMultiply/1
  Mux/1 -> MatrixMultiply/2
  MatrixMultiply/1 -> Demux1/1

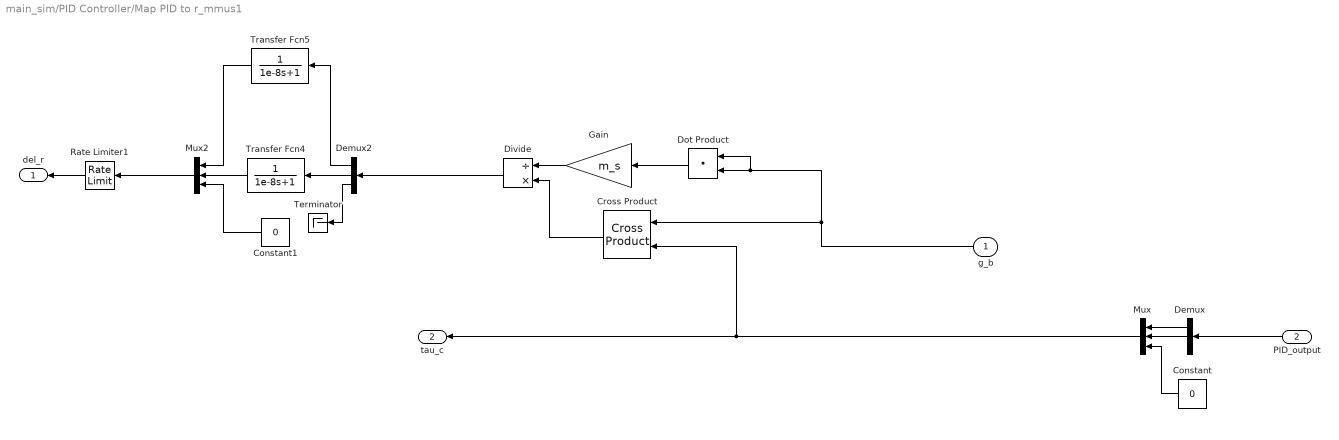
== system main_sim/PID Controller/Map PID to r_mmus1 ==
  g_b : Inport
  PID_output : Inport  Port=2
  Constant : Constant  Value=0
  Constant1 : Constant  Value=0
  Cross Product : matrix_library/Cross Product
  Demux : Demux  Outputs=3
  Demux2 : Demux  Outputs=3
  Divide : Product  Inputs=/*
  Dot Product : DotProduct  OutDataTypeStr=Inherit: Inherit via internal rule
  Gain : Gain  Gain=m_s
  Mux : Mux  Inputs=3
  Mux2 : Mux  Inputs=3
  Rate Limiter1 : RateLimiter  RisingSlewLimit=0.030  FallingSlewLimit=-0.030  SampleTimeMode=inherited
  Terminator : Terminator
  Transfer Fcn4 : TransferFcn  Denominator=[1e-8 1]
  Transfer Fcn5 : TransferFcn  Denominator=[1e-8 1]
  del_r : Outport
  tau_c : Outport  Port=2
  wires:
  PID_output/1 -> Demux/1
  g_b/1 -> Dot Product/1, Dot Product/2, Cross Product/1
  Demux/2 -> Mux/2
  Demux/1 -> Mux/1
  Constant/1 -> Mux/3
  Mux/1 -> Cross Product/2, tau_c/1
  Dot Product/1 -> Gain/1
  Gain/1 -> Divide/1
  Cross Product/1 -> Divide/2
  Transfer Fcn4/1 -> Mux2/2
  Constant1/1 -> Mux2/3
  Transfer Fcn5/1 -> Mux2/1
  Divide/1 -> Demux2/1
  Mux2/1 -> Rate Limiter1/1
  Demux2/2 -> Transfer Fcn4/1
  Demux2/1 -> Transfer Fcn5/1
  Rate Limiter1/1 -> del_r/1
  Demux2/3 -> Terminator/1

== system main_sim/PID Controller/PID Law ==
  P : Inport
  I : Inport  Port=2
  D : Inport  Port=3
  Gain : Gain  Gain=K_omega
  Gain1 : Gain  Gain=K_I
  Gain2 : Gain  Gain=K_q
  Gain3 : Gain  Gain=-1
  Sum : Sum  Inputs=|+++
  PID Output : Outport
  wires:
  Gain2/1 -> Sum/1
  P/1 -> Gain2/1
  Gain/1 -> Sum/3
  D/1 -> Gain/1
  Gain1/1 -> Sum/2
  I/1 -> Gain1/1
  Sum/1 -> Gain3/1
  Gain3/1 -> PID Output/1

== system main_sim/Plant Truth/quaternion to g_b, sanity check ==
  q_b_N : Inport
  Constant3 : Constant  Value=g_N
  Matrix Multiply : Product  Multiplication=Matrix(*)
  Quaternions to Direction Cosine Matrix : sharedtransform/Quaternions to  Direction Cosine Matrix  aMode=aMode
  g_b : Outport
  wires:
  Constant3/1 -> Matrix Multiply/2
  Quaternions to Direction Cosine Matrix/1 -> Matrix Multiply/1  "C_b_N"
  q_b_N/1 -> Quaternions to Direction Cosine Matrix/1
  Matrix Multiply/1 -> g_b/1  "g_b"

== system main_sim/Speed Control for LSR/Subsystem1 ==
  Mux1 : Mux  Inputs=3
  Sine Wave : Sin  Amplitude=h_d_amp_LSR(1)  Frequency=1/h_d_period_LSR(1)  Phase=h_d_phase_LSR(1)  SampleTime=0
  Sine Wave1 : Sin  Amplitude=h_d_amp_LSR(2)  Frequency=1/h_d_period_LSR(2)  Phase=h_d_phase_LSR(2)  SampleTime=0
  Sine Wave2 : Sin  Amplitude=h_d_amp_LSR(3)  Frequency=1/h_d_period_LSR(3)  Phase=h_d_phase_LSR(3)  SampleTime=0
  h_d : Outport
  wires:
  Sine Wave/1 -> Mux1/1
  Sine Wave2/1 -> Mux1/3
  Sine Wave1/1 -> Mux1/2
  Mux1/1 -> h_d/1

== system main_sim/Speed Control for LSR/Subsystem2 ==
  Gain : Gain  Gain=1/h_d_period(1)
  Gain1 : Gain  Gain=1/h_d_period(2)
  Gain2 : Gain  Gain=1/h_d_period(3)
  Mux : Mux  Inputs=3
  Sine Wave3 : Sin  Amplitude=h_d_amp_LSR(1)  Frequency=1/h_d_period_LSR(1)  Phase=h_d_phase_LSR(1)-(pi/2)  SampleTime=0
  Sine Wave4 : Sin  Amplitude=h_d_amp_LSR(2)  Frequency=1/h_d_period_LSR(2)  Phase=h_d_phase_LSR(2)-(pi/2)  SampleTime=0
  Sine Wave5 : Sin  Amplitude=h_d_amp_LSR(3)  Frequency=1/h_d_period_LSR(3)  Phase=h_d_phase_LSR(3)-(pi/2)  SampleTime=0
  h_d_dot : Outport
  wires:
  Mux/1 -> h_d_dot/1
  Sine Wave5/1 -> Gain2/1
  Gain2/1 -> Mux/3
  Sine Wave3/1 -> Gain/1
  Sine Wave4/1 -> Gain1/1
  Gain1/1 -> Mux/2
  Gain/1 -> Mux/1

== matlab function main_sim/Extended Kalman Filter/Predict P ==
  data: F_k input; L input; Q input; P_kn1 input; P_k_min output
function P_k_min = predict_P(F_k,L,Q,P_kn1)

P_k_min = F_k*P_kn1*F_k' + L*Q*L';

end

== matlab function main_sim/Extended Kalman Filter/Predict Meausrements ==
  data: x_hat input; y_hat output
function y_hat = h(x_hat)

eta = x_hat(4);
eps = x_hat(5:7);

g_N = [0 0 -9.81]';

y_hat = [eta*eye(3)-skew(eps), -eps]*[ g_N, skew(g_N); 
                                   0     , -g_N']*[eta; eps];

== matlab function main_sim/UKF/CalcSigmaPoints1 ==
  data: x_kn1 input; x_kn1_i output; P_kn1 input; Wm output; Wc output; flag output
function [x_kn1_i,Wm,Wc,flag] = calc_sigma_points(x_kn1, P_kn1)

n = size(x_kn1,1);

alpha   = 1e-3;         % small, positive
kappa   = 0;            % usually 0
beta    = 2;            % optimal for Gaussian

alpha = 1e-2;           % or 1e-1 to start
kappa = 3 - n;          % common choice
beta  = 2;

lambda  = alpha^2*(n+kappa) - n;

P_kn1 = 0.5*(P_kn1 + P_kn1.');         % symmetrize
scl = (n + lambda);
if scl <= 0, error('n+lambda must be > 0'); end
[root,flag] = chol(scl*(P_kn1 + 1e-12*eye(n)), 'lower');
if flag>0
    % escalate jitter if needed
    for k = 1:5
        [root,flag] = chol(scl*(P_kn1 + 10^(k-12)*eye(n)), 'lower');
        if flag==0, break; end
    end
    if flag>0
        error('P_kn1 is not SPD at this step (even with jitter).');
    end
end

x_kn1_i = zeros(n,2*n + 1);
x_kn1_i(:,1) = x_kn1; % central point

for i = 1:n
    x_kn1_i(:,i+1)   = x_kn1 + root(:,i);
    x_kn1_i(:,i+1+n) = x_kn1 - root(:,i);
end
      

Wm      = 0.5 /(n+lambda) * ones(2*n+1,1);
Wc      = Wm;
Wm(1)   = lambda/(n+lambda);
Wc(1)   = Wm(1) + (1-alpha^2+beta);

== matlab function main_sim/Extended Kalman Filter/Calculate H ==
  data: x input; H output
function H = calc_H(x)
% x = [omega(3); eta; eps(3)]
% omega = x(1:3); 
eta   = x(4);
eps  = x(5:7);

g_N = [0;0;-9.81];
g_N_hat  = g_N / norm(g_N);


H_omega = zeros(3,3);
H_eta   = 2*(eta*eye(3) - skew(eps))*g_N_hat;               % 3x1
H_eps   = 2*((eps.'*g_N_hat)*eye(3) + eps*g_N_hat.' - g_N_hat*eps.' + eta*skew(g_N_hat));  % 3x3

H = [H_omega, H_eta, H_eps];
end

== matlab function main_sim/UKF/Correct ==
  data: y_k input; y_hat_k input; P_y input; P_xy input; x_k_minus input; x_k_plus output; P_k_minus input; P_k_plus output; sigma_r_z output
function [x_k_plus,P_k_plus,sigma_r_z] = correct(y_k, y_hat_k, P_y,P_xy,x_k_minus,P_k_minus)

K = P_xy/P_y;


x_k_plus = x_k_minus + K*(y_k-y_hat_k);
x_k_plus(4:7) = x_k_plus(4:7)./norm(x_k_plus(4:7));
P_k_plus = P_k_minus - K*P_y*K';

sigma_r_z = sqrt(P_k_plus(end,end));

== matlab function main_sim/UKF/Intermediate step: calculate P_y and P_xy ==
  data: y_hat_k input; y_k_i input; P_y output; x_k_i input; x_k_minus input; P_xy output; R input; Wc input
function [P_y,P_xy] = calc_Py_and_Px(y_hat_k,y_k_i,x_k_i,x_k_minus,R,Wc)

diff_y = y_k_i - y_hat_k;
diff_x = x_k_i - x_k_minus;

P_y = diff_y * diag(Wc) * diff_y' + R;
P_xy = diff_x * diag(Wc) * diff_y';

== matlab function main_sim/FSFB Controller/FSFB Quaternion Controller ==
  data: q_e input; omega input; tau_c output; Kp input; Kd input
function tau_c = fcn(q_e,omega,Kp,Kd)

q_e = q_e(:);
eta = q_e(1);
eps = q_e(2:4);

eps = eps(:);
omega = omega(:);
tau_c = -(Kp)*eps - Kd*omega;

== matlab function main_sim/UKF/Propagate State ==
  data: x_kn1_i input; x_k_i output; T input; J input; m_s input
function x_k_i = f(x_kn1_i,T,J,m_s)
    n = size(x_kn1_i,1);
    x_k_i = zeros(n,2*n+1);
    for i = 1:2*n+1
        omega_kn1 = x_kn1_i(1:3,i);
        eta_kn1 = x_kn1_i(4,i);
        eps_kn1 = x_kn1_i(5:7,i);

        q = [eta_kn1; eps_kn1;];
        % Gravity vector in body-frame
        g_b = [2*q(1)^2-1+2*q(2)^2 2*q(2)*q(3)-2*q(1)*q(4) 2*q(2)*q(4)+2*q(1)*q(3);
                2*q(2)*q(3)+2*q(1)*q(4) 2*q(1)^2-1+2*q(3)^2 2*q(3)*q(4)-2*q(1)*q(2);
                2*q(2)*q(4)-2*q(1)*q(3) 2*q(3)*q(4)+2*q(1)*q(2) 2*q(1)^2-1+2*q(4)^2]' * [0; 0; -9.81];

   
        r_z_kn1 = x_kn1_i(8,i);
        
        r_kn1 = [0 0 r_z_kn1]';
        
        x_k_i(:,i) = x_kn1_i(:,i) + T*[J\(-skew(omega_kn1)*J*omega_kn1 + m_s*skew(r_kn1)*g_b); 
                                     -.5*eps_kn1'*omega_kn1;
                                      .5*(eta_kn1*eye(3) + skew(eps_kn1))*omega_kn1; 
                                       0];
        
        % normalize the quaternion portion of the state
        x_k_i(4:7,i) = x_k_i(4:7,i)./norm(x_k_i(4:7,i)); 
    end
end

== matlab function main_sim/UKF/Predict Meausrements ==
  data: Wm input; y_hat_k output; y_k_i output; x_k_i input; H input
function [y_hat_k,y_k_i]   = predict_measurements(Wm,x_k_i,H)

y_k_i = H * x_k_i;

y_hat_k = y_k_i * Wm;

== matlab function main_sim/UKF/Predict State and Covariance ==
  data: x_k_i input; Wm input; Wc input; x_k_minus output; P_k_minus output; Q input
function [x_k_minus,P_k_minus] = predict_state_and_covariance(x_k_i,Wm,Wc,Q)

x_k_minus = x_k_i * Wm;  % weighted mean  (matrix‑vector product)
x_k_minus(4:7) = x_k_minus(4:7)./norm(x_k_minus(4:7));

P_k_minus = (x_k_i - x_k_minus)*diag(Wc) * (x_k_i - x_k_minus)'+ Q;

== matlab function main_sim/Extended Kalman Filter/Compute Kalman Gain ==
  data: H input; K output; P_k_min input; R input
function K = fcn(H,P_k_min,R)

W = H*P_k_min*H'+ R;
K = (P_k_min*H')/W;

== matlab function main_sim/Extended Kalman Filter/Correct ==
  data: r_k input; H input; K input; x_k output; P_k_min input; x_k_min input; R input; P_k output
function [x_k,P_k] = fcn(r_k,H,K,P_k_min,x_k_min,R)

x_k = x_k_min + K*r_k;

x_k(4:7) = x_k(4:7)./(norm(x_k(4:7)));

P_k = (eye(7) - K*H)*P_k_min*(eye(7) - K*H)' + K*R*K';

== matlab function main_sim/Extended Kalman Filter/Predict Meausrements1 ==
  data: x_k input; g_b_EKF output
function g_b_EKF = h(x_k)

eta = x_k(4);
eps = x_k(5:7);

g_N = [0 0 -9.81]';

g_N_hat = g_N;

g_b_EKF = [eta*eye(3)-skew(eps), -eps]*[ g_N_hat, skew(g_N_hat); 
                                   0     , -g_N_hat']*[eta; eps];

== matlab function main_sim/FSFB Controller/Quat Multiply ==
  data: q input; q_e output; q_d input
function q_e = fcn(q,q_d)

q_e = [q_d(1) -q_d(2) -q_d(3) -q_d(4);
       q_d(2)  q_d(1) -q_d(4)  q_d(3);
       q_d(3)  q_d(4)  q_d(1) -q_d(2);
       q_d(4) -q_d(3)  q_d(2)  q_d(1);]*q;

== matlab function main_sim/3-axis momentum tracking/MATLAB Function ==
  data: omega input; tau_c output; J input; h_d input; h_d_dot input; Kappa input; h_s output
function [tau_c,h_s] = fcn(omega,J,h_d,h_d_dot,Kappa)
 
h_s = J*omega; % for plotting

tau_c = -Kappa*(h_s-h_d)+skew(omega)*h_s + h_d_dot;

== matlab function main_sim/Plant Truth/MATLAB Function ==
  data: omega input; r_0 input; m_s input; J input; tau input; del_r input; h_wheels input; omegadot output; q input; qdot output; eulerdot output; r output; euler input; g_b output; tau_g output
function [omegadot, qdot,eulerdot,r,g_b,tau_g] = fcn(omega,r_0,m_s,J,tau,del_r,h_wheels,q,euler)
% Equations of motion developed in the work of Chesi.

g = 9.81; % 

% Gravity vector in body-frame
C_N_b = [2*q(1)^2-1+2*q(2)^2 2*q(2)*q(3)-2*q(1)*q(4) 2*q(2)*q(4)+2*q(1)*q(3);
       2*q(2)*q(3)+2*q(1)*q(4) 2*q(1)^2-1+2*q(3)^2 2*q(3)*q(4)-2*q(1)*q(2);
       2*q(2)*q(4)-2*q(1)*q(3) 2*q(3)*q(4)+2*q(1)*q(2) 2*q(1)^2-1+2*q(4)^2];

eta = q(1);
eps = q(2:4);
C_b_N = (eta^2 - eps'*eps)*eye(3) + 2*(eps*eps') - 2*eta*skew(eps);

% g_b = C_N_b' * [0; 0; -g];
g_b = C_b_N* [0 0 -g]';

% Equations of Motion
omegadot=J\(-(cross(omega,J*omega) + cross(omega,h_wheels))+cross((r_0+del_r),g_b*m_s)+tau);
% tau_g = cross(r_0,g_b*m_s)-tau;
tau_g = m_s*cross((r_0),g_b);
r = (r_0 + del_r);

% Quaternion rates
qdot = 0.5*[0 -omega(1) -omega(2) -omega(3);
             omega(1) 0 omega(3) -omega(2);
             omega(2) -omega(3) 0 omega(1);
             omega(3) omega(2) -omega(1) 0]*q;

% Euler rates
Phi = euler(1);
Theta = euler(2);
Psi = euler(3);

matrix = (1/cos(Theta)).*[cos(Theta) sin(Phi)*sin(Theta)  cos(Phi)*sin(Theta);
                              0          cos(Phi)*cos(Theta) -sin(Phi)*cos(Theta);
                              0          sin(Phi)             cos(Phi)];

product = matrix * omega;

dPhi = product(1);
dTheta = product(2);
dPsi = product(3);

eulerdot = [dPhi dTheta dPsi]';

== matlab function main_sim/3-axis momentum tracking/MATLAB Function1 ==
  data: omega input; g_b input; del_r_dot output; J input; h_d input; Gamma input; m_s input; debug output
function [del_r_dot,debug] = fcn(omega,g_b,J,h_d,Gamma,m_s)

h_s = J*omega;
del_r_dot =  -m_s * Gamma * ( skew(g_b) ) * (h_s - h_d);

debug = ( skew(g_b) ) * (h_s - h_d);

== matlab function main_sim/Reaction Wheel Subsystem/MATLAB Function ==
  data: wheel_speeds input; h_wheels output; I_wheel input; A_truth input
function h_wheels = fcn(wheel_speeds,I_wheel,A_truth)

h_wheels = [0 0 0]';
for i = 1:4
    h_wheels = h_wheels + I_wheel*wheel_speeds(i)*A_truth(:,i);
end

== matlab function main_sim/Speed Control for LSR/MATLAB Function ==
  data: omega input; tau_c output; J input; h_d input; h_d_dot input; Kappa input; h_s output
function [tau_c,h_s] = fcn(omega,J,h_d,h_d_dot,Kappa)
 
h_s = J*omega; % for plotting

tau_c = -Kappa*(h_s-h_d)+skew(omega)*h_s + h_d_dot;

== matlab function main_sim/PID Controller/MATLAB Function1 ==
  data: g_b input; P output
function P = fcn(g_b)

P = eye(3) - (g_b*g_b')/(norm(g_b)^2);

== matlab function main_sim/Estimator1/MATLAB Function1 ==
  data: omega_b input; g_b input; m_s input; gamma input; rhat_dot output; r_hat input
function rhat_dot = rhat_dot_adaptive(omega_b, g_b, m_s, gamma,r_hat)
%#codegen
% rhat_dot_adaptive  Adaptive law for r-hat-dot (Chesi)
% Inputs:
%   omega_b [3x1]  body rates (rad/s)
%   g_b     [3x1]  gravity vector in body frame (m/s^2)
%   m_s     [1x1]  total simulator mass (kg)
%   gamma   [1x1]  adaptation gain (>=0), use 1.0 for nominal
% Output:
%   rhat_dot [3x1] derivative of r-hat (m/s)

% Guards
if nargin < 4, gamma = 1.0; end
omega_b = reshape(omega_b,3,1);
g_b     = reshape(g_b,3,1);

% Chesi adaptive law:
% r_hat_dot = (m_s * g_b^x) * omega = m_s * (g_b x omega)
% Optional gamma lets you slow/speed adaptation for numerical robustness.

P_parr = (g_b*g_b')./(norm(g_b)^2);
rhat_dot = gamma * m_s * cross(g_b, omega_b);

end

== matlab function main_sim/Estimator1/MATLAB Function2 ==
  data: omega_b input; tau output; g_b input; rhat input; m_s input; k_p input; eps_g input; tau_max input; Pp output
function [tau,Pp] = tau_chesi(omega_b, g_b, rhat, m_s, k_p, eps_g, tau_max)
%#codegen
% tau_chesi  Control torque per Chesi
% Inputs:
%   omega_b [3x1]  body rates (rad/s)
%   g_b     [3x1]  gravity vector in body frame (m/s^2)
%   rhat    [3x1]  current estimate of r_0 (m)
%   m_s     [1x1]  total mass (kg)
%   k_p     [1x1]  positive gain
%   eps_g   [1x1]  small guard on ||g_b||^2 (e.g., 1e-8)
%   tau_max [1x1]  (optional) torque saturation (Nm); pass <=0 to disable
% Output:
%   tau [3x1] control torque (Nm)

if nargin < 6 || isempty(eps_g),  eps_g  = 1e-8; end
if nargin < 7 || isempty(tau_max), tau_max = 0;   end

omega_b = reshape(omega_b,3,1);
g_b     = reshape(g_b,3,1);
rhat    = reshape(rhat,3,1);

% Project omega onto the plane orthogonal to g_b:
gg   = g_b.'*g_b;
den  = max(gg, eps_g);
Pp   = eye(3) - (g_b*g_b.')/den;   % I - (g g^T)/||g||^2
omega_p = Pp * omega_b;

% Chesi control: tau = m_s * (g_b x rhat) - k_p * omega_p
tau = m_s * cross(g_b, rhat) - k_p * omega_p;

% Optional saturation for numerical stability in simulation
if tau_max > 0
    n = norm(tau);
    if n > tau_max
        tau = tau * (tau_max / n);
    end
end

end

== matlab function main_sim/Propagate Test/Propagate State ==
  data: x_kn1_i input; x_k_i output; T input; J input; m_s input
function x_k_i = f(x_kn1_i,T,J,m_s)
    omega_kn1 = x_kn1_i(1:3);
    eta_kn1 = x_kn1_i(4);
    eps_kn1 = x_kn1_i(5:7);
    r_z_kn1 = x_kn1_i(8);

    q = [eta_kn1; eps_kn1;];
    % Gravity vector in body-frame
    g_b = [2*q(1)^2-1+2*q(2)^2 2*q(2)*q(3)-2*q(1)*q(4) 2*q(2)*q(4)+2*q(1)*q(3);
            2*q(2)*q(3)+2*q(1)*q(4) 2*q(1)^2-1+2*q(3)^2 2*q(3)*q(4)-2*q(1)*q(2);
            2*q(2)*q(4)-2*q(1)*q(3) 2*q(3)*q(4)+2*q(1)*q(2) 2*q(1)^2-1+2*q(4)^2]' * [0; 0; -9.81];



    
    omega_kn1_cross = [0           -omega_kn1(3) omega_kn1(2);
                       omega_kn1(3) 0           -omega_kn1(1);
                      -omega_kn1(2) omega_kn1(1) 0];
    
    eps_kn1_cross = [0         -eps_kn1(3) eps_kn1(2);
                     eps_kn1(3) 0         -eps_kn1(1);
                    -eps_kn1(2) eps_kn1(1) 0];

    r_cross_g = [-r_z_kn1*g_b(2);
                  r_z_kn1*g_b(1);
                  0];
    
    x_k_i = x_kn1_i + T*[J\(-omega_kn1_cross*J*omega_kn1 + m_s*r_cross_g); 
                                 -.5*eps_kn1'*omega_kn1;
                                  .5*(eta_kn1*eye(3) + eps_kn1_cross)*omega_kn1; 
                                   0];
    
    % normalize the quaternion portion of the state
    x_k_i(4:7) = x_k_i(4:7)./norm(x_k_i(4:7)); 
end

== matlab function main_sim/PID Controller/Quat Multiply ==
  data: q input; q_e output; q_d input
function q_e = fcn(q,q_d)

q_e = [q_d(1) -q_d(2) -q_d(3) -q_d(4);
       q_d(2)  q_d(1) -q_d(4)  q_d(3);
       q_d(3)  q_d(4)  q_d(1) -q_d(2);
       q_d(4) -q_d(3)  q_d(2)  q_d(1);]*q;

== matlab function main_sim/IMU Model/Bias ==
  data: Tc input; sigma_x input; Ts input; x_prev input; b output; x_next output
function [b, x_next] = GM1_bias_model(Tc, sigma_x, Ts,x_prev)
% First-order Gauss–Markov bias, stateless (feedback via Unit Delay).

%   x_k = a x_{k-1} + w_k, where a = exp(-Ts/Tc)
%   Var{w_k} = sigma_x^2 * (1 - exp(-2*Ts/Tc))


% Exact discrete coefficient and driving-noise std 
a           = exp(-Ts ./ Tc);
sqrtVar_wk  = sqrt( (sigma_x.^2) .* (1 - exp(-2*Ts ./ Tc)) );

% Draw w_k and propagate
% rng('shuffle')
wk     = sqrtVar_wk .* randn(3,1);
x_next = a .* x_prev + wk;

% Bias output
b = x_next;   % same units as sigma_x (e.g., deg/s or rad/s)
end

== matlab function main_sim/IMU Model/Bias1 ==
  data: Tc input; sigma_x input; Ts input; x_prev input; b output; x_next output
function [b, x_next] = GM1_bias_model(Tc, sigma_x, Ts,x_prev)
% First-order Gauss–Markov bias, stateless (feedback via Unit Delay).

%   x_k = a x_{k-1} + w_k, where a = exp(-Ts/Tc)
%   Var{w_k} = sigma_x^2 * (1 - exp(-2*Ts/Tc))


% Exact discrete coefficient and driving-noise std 
a           = exp(-Ts ./ Tc);
sqrtVar_wk  = sqrt( (sigma_x.^2) .* (1 - exp(-2*Ts ./ Tc)) );

% Draw w_k and propagate
% rng('shuffle')
wk     = sqrtVar_wk .* randn(3,1);
x_next = a .* x_prev + wk;

% Bias output
b = x_next;   % same units as sigma_x (e.g., deg/s or rad/s)
end

== matlab function main_sim/Extended Kalman Filter/Propagate State ==
  data: x_kn1 input; omega_meas input; x_k_min output; T input; J input; tau_c input
function x_k_min = f(x_kn1,omega_meas,T,J,tau_c)
    % omega_kn1 = x_kn1(1:3);
    omega_kn1 = omega_meas;
    eta_kn1 = x_kn1(4);
    eps_kn1 = x_kn1(5:7);

    x_k_min = x_kn1 + T*[J\(-skew(omega_kn1)*J*omega_kn1+tau_c); 
                                 -.5*eps_kn1'*omega_kn1;
                                  .5*(eta_kn1*eye(3) + skew(eps_kn1))*omega_kn1;];

    x_k_min(1:3) = omega_meas;
    
end

== matlab function main_sim/Extended Kalman Filter/Calculate F ==
  data: x_k_min input; F output; T input; J input
function F = jacobian_f(x_k_min, T, J)

omega = x_k_min(1:3);
eta   = x_k_min(4);
eps  = x_k_min(5:7);

A11 = J \ (-skew(omega)*J + skew(J*omega));        % d(omegadot)/d(omega)
A12 = zeros(3,1);                       % d(omegadot)/d(eta)
A13 = zeros(3,3);                       % d(omegadot)/d(eps)

A21 = -0.5*eps.';                      % d(etadot)/d(omega)  (1x3)
A22 = 0;                                % d(etadot)/d(eta)
A23 = -0.5*omega.';                     % d(etadot)/d(eps)    (1x3)

A31 = 0.5*(eta*eye(3) + skew(eps));              % d(epsdot)/d(omega)  (3x3)
A32 = 0.5*omega;                        % d(epsdot)/d(eta)    (3x1)
A33 = -0.5*skew(omega);                         % d(epsdot)/d(eps)    (3x3)

A = [ A11  A12  A13;
      A21  A22  A23;
      A31  A32  A33 ];

F = eye(7) + T*A;

end
